simulink model "tv_system_lut"  (R2021b)
settings: Solver=VariableStepAuto  StartTime=0.0  StopTime=0  RelTol=1e-3
values from neighbouring files (symbols this model uses):
  gamma1 = 0.005    [main_pixloss.m]
  gamma2 = 1/(1.05*tau2)*(1/gamma1-beta/2)    [main_pixloss.m]
  lambda = 0.012    [main_pixloss.m]
  maxIter = 500    [main_pixloss.m]
  Np = 50    [main_pixloss.m]
undefined symbols (not defined in the file or in its folder): cols, gray, rows
libraries: visionsources x3, visionstatistics x2
(part 3 of 5)

== matlab function tv_system_lut/Subsystem1/For Iterator Subsystem1/Subsystem/MATLAB Function3 ==
  data: x input; out output; y input; div input
function out = l2_lut_noproduct(x,y,div)
x = min(max(x,-1),1);
y = min(max(y,-1),1);
divide_val = linspace(-1, 1, div);
[tmp1,tmp2] = meshgrid(divide_val);

truthtable = sqrt(tmp1.^2 + tmp2.^2);
truthtable = triu(truthtable);
vector_truthtable = truthtable(logical(truthtable));

% tmp1 = zeros(size(x));
% tmp2 = zeros(size(y));
truthtable_out_x = ones(size(x));
truthtable_out_y = ones(size(x));
for i = 1:numel(x)
    if x(i) < y(i)
        in_x = x(i);
        in_y = y(i);
    else
        in_x = y(i);
        in_y = x(i);
    end
    for k = 1:length(divide_val)
        if in_x > divide_val(k)
            truthtable_out_x(i) = k;
        end
        if in_y > divide_val(k)
            truthtable_out_y(i) = k;
        end
    end
end

out = cast(zeros(size(x)),'like',x);
for i = 1:numel(x)
    %out(i) = truthtable(div * truthtable_out_y(i)+truthtable_out_x(i));
    %out(i) = truthtable(truthtable_out_x(i),truthtable_out_y(i));

    n = truthtable_out_y(i);
    d = -1;
    a = div-1;
    zerosum = (1/2)*(n)*(2*a + (n-1)*(d));
    out(i) = vector_truthtable(div*truthtable_out_y(i) - zerosum + truthtable_out_x(i));
end
end

== matlab function tv_system_lut/For Iterator Subsystem2/For Iterator Subsystem/MATLAB Function ==
  data: error input; u input; erro output
function erro = fcn(error,u)

erro = norm(error(:),2) / norm(u(:),2);

== matlab function tv_system_lut/For Iterator Subsystem2/For Iterator Subsystem/MATLAB Function1 ==
  data: u input; y1 output; y2 output
function [y1,y2] = fcn(u)
    y1 = u(:,:,1);
    y2 = u(:,:,2);
end

== matlab function tv_system_lut/MATLAB Function ==
  data: res input; u input; mse output
function mse = fcn(res,u)

mse = immse(u,res);

== matlab function tv_system_lut/For Iterator Subsystem2/For Iterator Subsystem/MATLAB Function2 ==
  data: x input; tmp2 output; l2_x input
function tmp2 = fcn(x,l2_x)

if isfi(x) == true
    tmp2 = divide(x.numerictype,1,l2_x);
else
    tmp2 = 1./l2_x;
end

== matlab function tv_system_lut/MATLAB Function2 ==
  data: res input; u input; mse output
function mse = fcn(res,u)

mse = immse(u,res);

== matlab function tv_system_lut/For Iterator Subsystem2/For Iterator Subsystem/MATLAB Function3 ==
  data: tmp2 input; y output; lambda input; x input
function y = fcn(tmp2,lambda,x)

% tmp3 = lambda*tmp2;
y = repmat(max(1 - tmp2,0),1,1,2) .* x;

== matlab function tv_system_lut/For Iterator Subsystem2/For Iterator Subsystem/Subsystem/MATLAB Function ==
  data: in1 input; out output; in2 input
function out = abslut10(in1,in2)

divide_val = [ -1.0000000000000000000000000000000000000000000000000000000, -0.7777777777777776790912866999860852956771850585937500000, -0.5555555555555555802271783250034786760807037353515625000, -0.3333333333333333148296162562473909929394721984863281250, -0.1111111111111111049432054187491303309798240661621093750, 0.1111111111111111049432054187491303309798240661621093750, 0.3333333333333333148296162562473909929394721984863281250, 0.5555555555555555802271783250034786760807037353515625000, 0.7777777777777776790912866999860852956771850585937500000, 1.0000000000000000000000000000000000000000000000000000000,];

vector_truthtable = [1.4142135623730951454746218587388284504413604736328125000,1.2668615834434866496138738511945120990276336669921875000,1.0999438818457403232997648956370539963245391845703125000,1.1439589045541112000137218274176120758056640625000000000,0.9558139185602917420325752573262434452772140502929687500,0.7856742013183861672587227076292037963867187500000000000,1.0540925533894598409290210838662460446357727050781250000,0.8461970117626563814283713327313307672739028930664062500,0.6478835438717001071751155905076302587985992431640625000,0.4714045207910316781507731320743914693593978881835937500,1.0061539042374907371169001635280437767505645751953125000,0.7856742013183860562364202451135497540235519409179687500,0.5665577237325316595217827853048220276832580566406250000,0.3513641844631532618059566175361396744847297668457031250,0.1571348402636772167983991721484926529228687286376953125,1.0061539042374907371169001635280437767505645751953125000,0.7856742013183860562364202451135497540235519409179687500,0.5665577237325316595217827853048220276832580566406250000,0.3513641844631532618059566175361396744847297668457031250,0.1571348402636772167983991721484926529228687286376953125,0.1571348402636772167983991721484926529228687286376953125,1.0540925533894598409290210838662460446357727050781250000,0.8461970117626563814283713327313307672739028930664062500,0.6478835438717001071751155905076302587985992431640625000,0.4714045207910316781507731320743914693593978881835937500,0.3513641844631532618059566175361396744847297668457031250,0.3513641844631532618059566175361396744847297668457031250,0.4714045207910316781507731320743914693593978881835937500,1.1439589045541112000137218274176120758056640625000000000,0.9558139185602917420325752573262434452772140502929687500,0.7856742013183861672587227076292037963867187500000000000,0.6478835438717001071751155905076302587985992431640625000,0.5665577237325316595217827853048220276832580566406250000,0.5665577237325316595217827853048220276832580566406250000,0.6478835438717001071751155905076302587985992431640625000,0.7856742013183861672587227076292037963867187500000000000,1.2668615834434866496138738511945120990276336669921875000,1.0999438818457403232997648956370539963245391845703125000,0.9558139185602917420325752573262434452772140502929687500,0.8461970117626563814283713327313307672739028930664062500,0.7856742013183860562364202451135497540235519409179687500,0.7856742013183860562364202451135497540235519409179687500,0.8461970117626563814283713327313307672739028930664062500,0.9558139185602917420325752573262434452772140502929687500,1.0999438818457403232997648956370539963245391845703125000,1.4142135623730951454746218587388284504413604736328125000,1.2668615834434866496138738511945120990276336669921875000,1.1439589045541112000137218274176120758056640625000000000,1.0540925533894598409290210838662460446357727050781250000,1.0061539042374907371169001635280437767505645751953125000,1.0061539042374907371169001635280437767505645751953125000,1.0540925533894598409290210838662460446357727050781250000,1.1439589045541112000137218274176120758056640625000000000,1.2668615834434866496138738511945120990276336669921875000,1.4142135623730951454746218587388284504413604736328125000,];

div = 10;

if in1 < in2
    in_x = in1;
    in_y = in2;
else
    in_x = in2;
    in_y = in1;
end

logical_x = (in_x >= divide_val);
logical_y = (in_y >= divide_val);

truthtable_out_x = nnz(logical_x);
truthtable_out_y = nnz(logical_y);

n = truthtable_out_y;
d = -1;
a = div-1;
zerosum = (1/2)*(n)*(2*a + (n-1)*(d));
out = vector_truthtable(div*truthtable_out_y - zerosum + truthtable_out_x);


end
